simulink model "LabFD_OLFreqResponse"  (R2016a)
settings: Solver=VariableStepAuto  StartTime=0.0  StopTime=30  MaxStep=.005  RelTol=1e-3
settings Model: Creator=jordan  LastModifiedBy=jordan

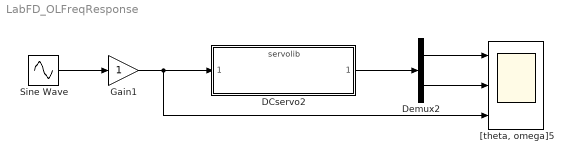
== system LabFD_OLFreqResponse ==
  DCservo2 : ModelReference  ModelNameDialog=servolib.slx  SimulationMode=Normal  ModelReferenceVersion=1.70
  Demux2 : Demux  Outputs=2
  Gain1 : Gain
  Sine Wave : Sin  Frequency=50  SampleTime=0
  "[theta, omega]5" : Scope  NumInputPorts=3
  wires:
  DCservo2/1 -> Demux2/1
  Demux2/2 -> "[theta, omega]5"/2
  Demux2/1 -> "[theta, omega]5"/1
  Sine Wave/1 -> Gain1/1
  Gain1/1 -> "[theta, omega]5"/3, DCservo2/1
